simulink model "final_model16b"  (Simulink 8.8)
settings: Solver=ode5  StartTime=0.0  StopTime=0.8  FixedStep=1e-06  RelTol=1e-3
undefined symbols (not defined in the file or in its folder): Acid, Lead
libraries: spsCurrentMeasurementLib x14, spsSeriesRLCBranchLib x12, simulink x9, spsVoltageMeasurementLib x9, spsIGBTDiodeLib x6, spsDiodeLib x5, spsParallelRLCBranchLib x4, spsMosfetLib x2, spsAlphaBetaZerotodq0Lib x2, spsBatteryLib x1, spspowerguiLib x1, spsThreePhaseVIMeasurementLib x1
settings Model: Creator=Aditya  LastModifiedBy=Aditya
settings DataIOCC: LimitDataPoints=off  SaveFormat=Dataset  SignalLoggingSaveFormat=Dataset  ReturnWorkspaceOutputs=on
settings OptimizationCC: LifeSpan=auto
settings DebuggingCC: UnderspecifiedInitializationDetection=Simplified  MergeDetectMultiDrivingBlocksExec=error  FcnCallInpInsideContextMsg=error  StateNameClashWarn=none  SFUnexpectedBacktrackingDiag=error  SFNoUnconditionalDefaultTransitionDiag=error  SFExecutionAtInitializationDiag=warning  SFMachineParentedDataDiag=error
settings HardwareCC: ProdBitPerPointer=64  ProdBitPerSizeT=64  ProdBitPerPtrDiffT=64  ProdLargestAtomicFloat=Float  ProdIntDivRoundTo=Zero  ProdEndianess=LittleEndian  ProdWordSize=64  ProdHWDeviceType=Intel->x86-64 (Windows64)
settings ModelReferenceCC: PropagateSignalLabelsOutOfModel=on
settings SFSimCC: SimUseLocalCustomCode=on
settings RTWCC: RTWUseLocalCustomCode=on
settings GRTTargetCC: TargetLangStandard=C99 (ISO)  CombineOutputUpdateFcns=on  GRTInterface=off
settings ConfigComp: CovMetricSettings=dwe  CovSaveCumulativeToWorkspaceVar=off  CovSaveSingleToWorkspaceVar=off  CovExternalEMLEnable=on

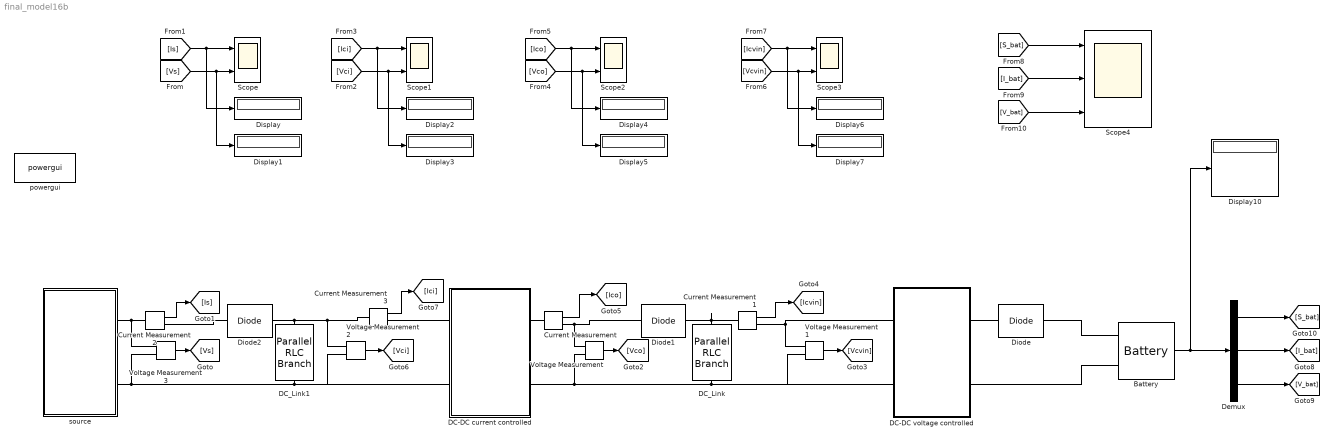
== system final_model16b ==
  Battery : spsBatteryLib/Battery  BatType=Lead-Acid  ShowTempParam=off  ThermalPreset=no  ShowAgeParam=off  NomV=48  NomQ=150  SOC=50  Batt_Tr=0.1  PresetModel=on  MaxQ=156.25  MinV=36  FullV=52.2632  Dis_rate=30  R=0.0032  Normal_OP=46.5417  expZone="[48.8684          0.5]"  current=[6.5 13 32.5]  Units=Time  Tci=20  NomT=20  T2=-30  MaxQ2=4.8  FullV2=7.1  Normal_OP2=5.655  expZone2="[6.58           1]"  Rca=0.6  ti=2000  Dp=0  Neq0=0  Tsim=1e6  Ta1=25  Qeol=5.4*0.9  Reol=0.013333*1.2  Char_age=[2.3478, 3]  Dis_age=[2.3478, 10]  N1=1500  N2=10500  N3=1000  N4=1400  Ta2=45  N5=950
  Current Measurement{,1..3} (4 alike) : spsCurrentMeasurementLib/Current Measurement  PhasorSimulation=off  OutputType=Complex  PSBequivalent=0
  DC-DC current controlled : Subsystem
  DC-DC voltage controlled : Subsystem
  DC_Link : spsParallelRLCBranchLib/Parallel RLC Branch  LConnTagsString=a  RConnTagsString=__new0  BranchType=C  Resistance=1  Inductance=1e-3  SetiL0=off  InitialCurrent=0  Capacitance=300e-6  Setx0=off  InitialVoltage=0  Measurements=None
  DC_Link1 : spsParallelRLCBranchLib/Parallel RLC Branch  LConnTagsString=a  RConnTagsString=__new0  BranchType=C  Resistance=1  Inductance=1e-3  SetiL0=off  InitialCurrent=0  Capacitance=300e-6  Setx0=off  InitialVoltage=0  Measurements=None
  Demux : Demux  Outputs=3
  Diode : spsDiodeLib/Diode  Ron=0.001  Lon=0  Vf=0.8  IC=0  UseSnubber=0  Rs=500  Cs=250e-9  Measurements=off
  Diode1 : spsDiodeLib/Diode  Ron=0.001  Lon=0  Vf=0.8  IC=0  UseSnubber=0  Rs=500  Cs=250e-9  Measurements=off
  Diode2 : spsDiodeLib/Diode  Ron=0.001  Lon=0  Vf=0.8  IC=0  UseSnubber=0  Rs=500  Cs=250e-9  Measurements=off
  Display{,1..7,10} (9 alike) : Display
  Scope{,1..3} (4 alike) : Scope  NumInputPorts=2
  Scope4 : Scope  NumInputPorts=3
  Voltage Measurement{,1..3} (4 alike) : spsVoltageMeasurementLib/Voltage Measurement  PhasorSimulation=off  OutputType=Complex  PSBequivalent=0
  powergui : spspowerguiLib/powergui  Priority=1  SimulationMode=Discrete  SampleTime=1e-06  frequency=60  Iterations=50  frequencyindice=0  Pbase=100e6  ErrMax=1e-4  UnitsV=kV  UnitsW=MW  buscounter=0  FunctionMessages=off  echomessages=off  EnableUseOfTLC=off  CurrentSourceSwitches=off  DisableSnubberDevices=off  DisableRonSwitches=off  DisableVfSwitches=off  DisplayEquations=off  AutomaticDiscreteSolvers=off  SolverType=Tustin/Backward Euler (TBE)  Interpol=off  ExternalGateDelay=off  methode=off  Ts=100  x0status=blocks  SPID=on  SwTol=0  HookPort=off  NonlinearTolerance=1e-4  nMaxIteration=100  ContinueOnMaxIteration=off  RestoreLinks=warning  ResistiveCurrentMeasurement=off  Frange=[0:2:500]  Ylog=off  Xlog=on  ShowGrid=off  save=off  variable=ZData  structure=0  ZoomFFT=off  StartTime=0.0  cycles=1  DisplayStyle=1  fundamental=60  FreqAxis=off  MaxFrequency=1000  frequencyindicesteady=1  RmsSteady=1  display=off
  source : Subsystem
  wires:
  Voltage Measurement3/1 -> [Vs]
  Current Measurement2/1 -> [Is]
  Voltage Measurement/1 -> [Vco]
  Voltage Measurement1/1 -> [Vcvin]
  Current Measurement/1 -> [Ico]
  Current Measurement1/1 -> [Icvin]
  Voltage Measurement2/1 -> [Vci]
  Current Measurement3/1 -> [Ici]
  [Is] -> Display/1, Scope/1
  [Vs] -> Display1/1, Scope/2
  [Vci] -> Display3/1, Scope1/2
  [Ici] -> Display2/1, Scope1/1
  [Vco] -> Display5/1, Scope2/2
  [Ico] -> Display4/1, Scope2/1
  [Vcvin] -> Display7/1, Scope3/2
  [Icvin] -> Display6/1, Scope3/1
  Battery/1 -> Demux/1, Display10/1
  Demux/1 -> [S_bat]
  Demux/2 -> [I_bat]
  Demux/3 -> [V_bat]
  [S_bat] -> Scope4/1
  [I_bat] -> Scope4/2
  [V_bat] -> Scope4/3
  connections:
  Current Measurement3/LConn1 -- Diode2/RConn1 -- DC_Link1/LConn1 -- Voltage Measurement2/LConn1
  source/LConn2 -- Voltage Measurement3/LConn2 -- Voltage Measurement2/LConn2 -- DC-DC current controlled/LConn2 -- DC_Link1/RConn1
  Current Measurement/RConn1 -- Diode1/LConn1 -- Voltage Measurement/LConn1
  DC-DC current controlled/RConn2 -- Voltage Measurement/LConn2 -- Voltage Measurement1/LConn2 -- DC-DC voltage controlled/LConn2 -- DC_Link/RConn1
  Current Measurement/LConn1 -- DC-DC current controlled/RConn1
  Voltage Measurement1/LConn1 -- Current Measurement1/RConn1 -- DC-DC voltage controlled/LConn1
  Current Measurement3/RConn1 -- DC-DC current controlled/LConn1
  Current Measurement2/LConn1 -- Voltage Measurement3/LConn1 -- source/LConn1
  Diode/LConn1 -- DC-DC voltage controlled/RConn1
  Battery/LConn2 -- DC-DC voltage controlled/RConn2
  Battery/LConn1 -- Diode/RConn1
  DC_Link/LConn1 -- Diode1/RConn1 -- Current Measurement1/LConn1
  Current Measurement2/RConn1 -- Diode2/LConn1

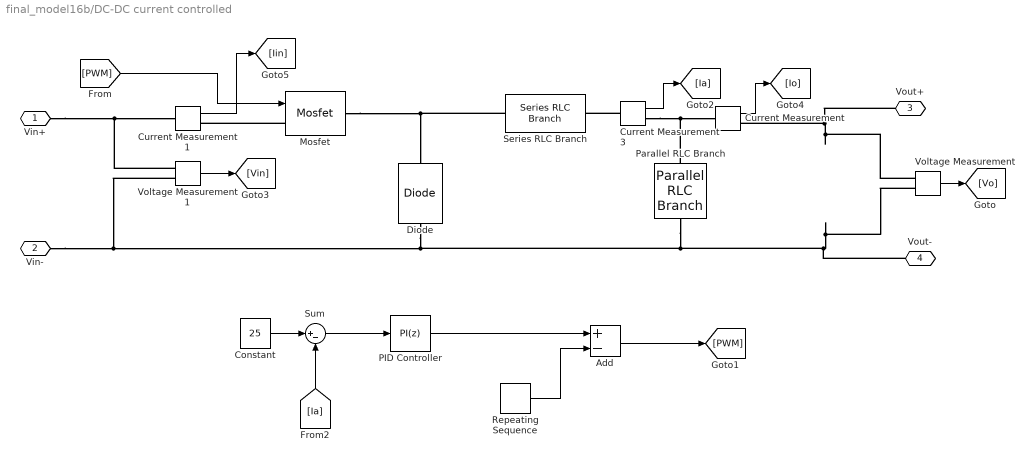
== system final_model16b/DC-DC current controlled ==
  Add : Sum  Inputs=+-
  Constant : Constant  Value=25
  Current Measurement : spsCurrentMeasurementLib/Current Measurement  PhasorSimulation=off  OutputType=Complex  PSBequivalent=0
  Current Measurement1 : spsCurrentMeasurementLib/Current Measurement  PhasorSimulation=off  OutputType=Complex  PSBequivalent=0
  Current Measurement3 : spsCurrentMeasurementLib/Current Measurement  PhasorSimulation=off  OutputType=Complex  PSBequivalent=0
  Diode : spsDiodeLib/Diode  Ron=0.001  Lon=0  Vf=0.8  IC=0  UseSnubber=0  Rs=500  Cs=250e-9  Measurements=off
  Mosfet : spsMosfetLib/Mosfet  Ron=0.1  Lon=0  Rd=0.01  Vfd=0  IC=0  Rs=1e5  Cs=inf  Measurements=off
  PID Controller : simulink/Continuous/PID Controller  Controller=PI  Form=Parallel  TimeDomain=Discrete-time  SampleTime=-1  IntegratorMethod=Forward Euler  ControllerParametersSource=internal  P=0.4928  I=0.93  D=0  UseFilter=on  N=100  InitialConditionSource=internal  InitialConditionForIntegrator=0  InitialConditionForFilter=0  DifferentiatorICPrevScaledInput=0  ExternalReset=none  TrackingMode=off  Kt=1  LimitOutput=off  UpperSaturationLimit=inf  LowerSaturationLimit=-inf  LinearizeAsGain=on  AntiWindupMode=none  Kb=1  POutMin=[]  POutMax=[]  IOutMin=[]  IOutMax=[]  DOutMin=[]  DOutMax=[]  NOutMin=[]  NOutMax=[]  SumOutMin=[]  SumOutMax=[]  SaturationOutMin=[]  SaturationOutMax=[]  PParamMin=[]  PParamMax=[]  IParamMin=[]  IParamMax=[]  DParamMin=[]  DParamMax=[]  NParamMin=[]  NParamMax=[]  KbParamMin=[]  KbParamMax=[]  KtParamMin=[]  KtParamMax=[]  KbOutMin=[]  KbOutMax=[]  KtOutMin=[]  KtOutMax=[]  IntegratorOutMin=[]  IntegratorOutMax=[]  FilterOutMin=[]  FilterOutMax=[]  SumI1OutMin=[]  SumI1OutMax=[]  SumI2OutMin=[]  SumI2OutMax=[]  SumI3OutMin=[]  SumI3OutMax=[]  SumDOutMin=[]  SumDOutMax=[]  DifferentiatorOutMin=[]  DifferentiatorOutMax=[]  IntegratorContinuousStateAttributes=''  IntegratorStateMustResolveToSignalObject=off  IntegratorRTWStateStorageClass=Auto  FilterContinuousStateAttributes=''  FilterStateMustResolveToSignalObject=off  FilterRTWStateStorageClass=Auto
  Parallel RLC Branch : spsParallelRLCBranchLib/Parallel RLC Branch  LConnTagsString=a  RConnTagsString=__new0  BranchType=C  Resistance=1  Inductance=1e-3  SetiL0=off  InitialCurrent=0  Capacitance=20e-6  Setx0=off  InitialVoltage=0  Measurements=None
  Repeating Sequence : simulink/Sources/Repeating Sequence  rep_seq_t=[0 0.25/2000 0.5/2000 0.75/2000 1/2000]  rep_seq_y=[0 -1 0 1 0]
  Series RLC Branch : spsSeriesRLCBranchLib/Series RLC Branch  LConnTagsString=__new0  RConnTagsString=__new0  BranchType=L  Resistance=10  Inductance=0.01  SetiL0=off  InitialCurrent=0  Capacitance=1e-6  Setx0=off  InitialVoltage=0  Measurements=None
  Sum : Sum  Inputs=|+-
  Voltage Measurement : spsVoltageMeasurementLib/Voltage Measurement  PhasorSimulation=off  OutputType=Complex  PSBequivalent=0
  Voltage Measurement1 : spsVoltageMeasurementLib/Voltage Measurement  PhasorSimulation=off  OutputType=Complex  PSBequivalent=0
  Vin+ : PMIOPort  Side=Left
  Vin- : PMIOPort  Port=2  Side=Left
  Vout+ : PMIOPort  Port=3  Side=Right
  Vout- : PMIOPort  Port=4  Side=Right
  wires:
  Sum/1 -> PID Controller/1
  Voltage Measurement1/1 -> [Vin]
  [PWM] -> Mosfet/1
  Constant/1 -> Sum/1
  PID Controller/1 -> Add/1
  Add/1 -> [PWM]
  Repeating Sequence/1 -> Add/2
  [Ia] -> Sum/2
  Current Measurement3/1 -> [Ia]
  Voltage Measurement/1 -> [Vo]
  Current Measurement/1 -> [Io]
  Current Measurement1/1 -> [Iin]
  connections:
  Mosfet/RConn1 -- Diode/RConn1 -- Series RLC Branch/LConn1
  Voltage Measurement1/LConn2 -- Vin-/RConn1 -- Voltage Measurement/LConn2 -- Vout-/RConn1 -- Parallel RLC Branch/RConn1 -- Diode/LConn1
  Parallel RLC Branch/LConn1 -- Current Measurement/LConn1 -- Current Measurement3/RConn1
  Mosfet/LConn1 -- Current Measurement1/RConn1
  Vout+/RConn1 -- Current Measurement/RConn1 -- Voltage Measurement/LConn1
  Voltage Measurement1/LConn1 -- Vin+/RConn1 -- Current Measurement1/LConn1
  Current Measurement3/LConn1 -- Series RLC Branch/RConn1

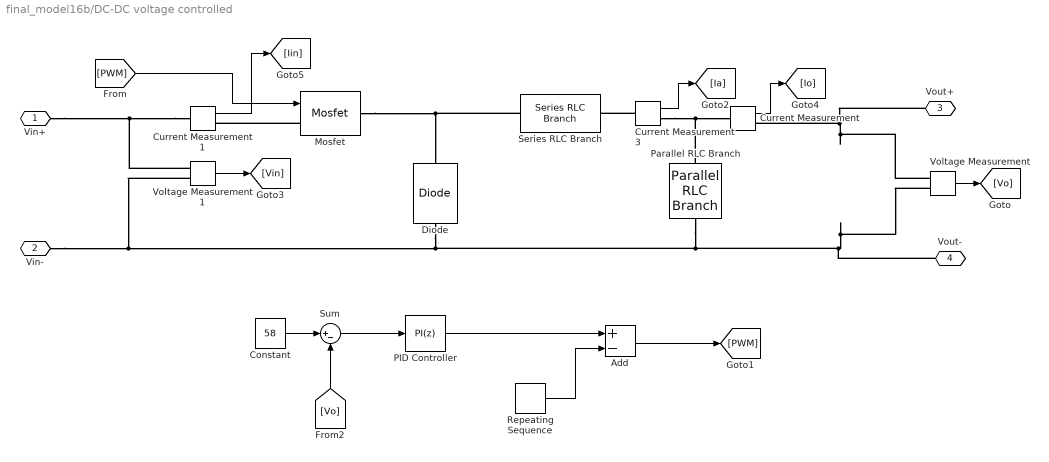
== system final_model16b/DC-DC voltage controlled ==
  Add : Sum  Inputs=+-
  Constant : Constant  Value=58
  Current Measurement : spsCurrentMeasurementLib/Current Measurement  PhasorSimulation=off  OutputType=Complex  PSBequivalent=0
  Current Measurement1 : spsCurrentMeasurementLib/Current Measurement  PhasorSimulation=off  OutputType=Complex  PSBequivalent=0
  Current Measurement3 : spsCurrentMeasurementLib/Current Measurement  PhasorSimulation=off  OutputType=Complex  PSBequivalent=0
  Diode : spsDiodeLib/Diode  Ron=0.001  Lon=0  Vf=0.8  IC=0  UseSnubber=0  Rs=500  Cs=250e-9  Measurements=off
  Mosfet : spsMosfetLib/Mosfet  Ron=0.1  Lon=0  Rd=0.01  Vfd=0  IC=0  Rs=1e5  Cs=inf  Measurements=off
  PID Controller : simulink/Continuous/PID Controller  Controller=PI  Form=Parallel  TimeDomain=Discrete-time  SampleTime=-1  IntegratorMethod=Forward Euler  ControllerParametersSource=internal  P=0.4928  I=0.93  D=0  UseFilter=on  N=100  InitialConditionSource=internal  InitialConditionForIntegrator=0  InitialConditionForFilter=0  DifferentiatorICPrevScaledInput=0  ExternalReset=none  TrackingMode=off  Kt=1  LimitOutput=off  UpperSaturationLimit=inf  LowerSaturationLimit=-inf  LinearizeAsGain=on  AntiWindupMode=none  Kb=1  POutMin=[]  POutMax=[]  IOutMin=[]  IOutMax=[]  DOutMin=[]  DOutMax=[]  NOutMin=[]  NOutMax=[]  SumOutMin=[]  SumOutMax=[]  SaturationOutMin=[]  SaturationOutMax=[]  PParamMin=[]  PParamMax=[]  IParamMin=[]  IParamMax=[]  DParamMin=[]  DParamMax=[]  NParamMin=[]  NParamMax=[]  KbParamMin=[]  KbParamMax=[]  KtParamMin=[]  KtParamMax=[]  KbOutMin=[]  KbOutMax=[]  KtOutMin=[]  KtOutMax=[]  IntegratorOutMin=[]  IntegratorOutMax=[]  FilterOutMin=[]  FilterOutMax=[]  SumI1OutMin=[]  SumI1OutMax=[]  SumI2OutMin=[]  SumI2OutMax=[]  SumI3OutMin=[]  SumI3OutMax=[]  SumDOutMin=[]  SumDOutMax=[]  DifferentiatorOutMin=[]  DifferentiatorOutMax=[]  IntegratorContinuousStateAttributes=''  IntegratorStateMustResolveToSignalObject=off  IntegratorRTWStateStorageClass=Auto  FilterContinuousStateAttributes=''  FilterStateMustResolveToSignalObject=off  FilterRTWStateStorageClass=Auto
  Parallel RLC Branch : spsParallelRLCBranchLib/Parallel RLC Branch  LConnTagsString=a  RConnTagsString=__new0  BranchType=C  Resistance=1  Inductance=1e-3  SetiL0=off  InitialCurrent=0  Capacitance=20e-6  Setx0=off  InitialVoltage=0  Measurements=None
  Repeating Sequence : simulink/Sources/Repeating Sequence  rep_seq_t=[0 0.25/2000 0.5/2000 0.75/2000 1/2000]  rep_seq_y=[0 -1 0 1 0]
  Series RLC Branch : spsSeriesRLCBranchLib/Series RLC Branch  LConnTagsString=__new0  RConnTagsString=__new0  BranchType=L  Resistance=10  Inductance=0.01  SetiL0=off  InitialCurrent=0  Capacitance=1e-6  Setx0=off  InitialVoltage=0  Measurements=None
  Sum : Sum  Inputs=|+-
  Voltage Measurement : spsVoltageMeasurementLib/Voltage Measurement  PhasorSimulation=off  OutputType=Complex  PSBequivalent=0
  Voltage Measurement1 : spsVoltageMeasurementLib/Voltage Measurement  PhasorSimulation=off  OutputType=Complex  PSBequivalent=0
  Vin+ : PMIOPort  Side=Left
  Vin- : PMIOPort  Port=2  Side=Left
  Vout+ : PMIOPort  Port=3  Side=Right
  Vout- : PMIOPort  Port=4  Side=Right
  wires:
  Constant/1 -> Sum/1
  Repeating Sequence/1 -> Add/2
  Current Measurement/1 -> [Io]
  Add/1 -> [PWM]
  PID Controller/1 -> Add/1
  [PWM] -> Mosfet/1
  Voltage Measurement/1 -> [Vo]
  Current Measurement3/1 -> [Ia]
  [Vo] -> Sum/2
  Sum/1 -> PID Controller/1
  Voltage Measurement1/1 -> [Vin]
  Current Measurement1/1 -> [Iin]
  connections:
  Current Measurement3/LConn1 -- Series RLC Branch/RConn1
  Mosfet/RConn1 -- Diode/RConn1 -- Series RLC Branch/LConn1
  Current Measurement3/RConn1 -- Current Measurement/LConn1 -- Parallel RLC Branch/LConn1
  Vout+/RConn1 -- Current Measurement/RConn1 -- Voltage Measurement/LConn1
  Diode/LConn1 -- Vin-/RConn1 -- Voltage Measurement1/LConn2 -- Voltage Measurement/LConn2 -- Vout-/RConn1 -- Parallel RLC Branch/RConn1
  Current Measurement1/LConn1 -- Vin+/RConn1 -- Voltage Measurement1/LConn1
  Mosfet/LConn1 -- Current Measurement1/RConn1

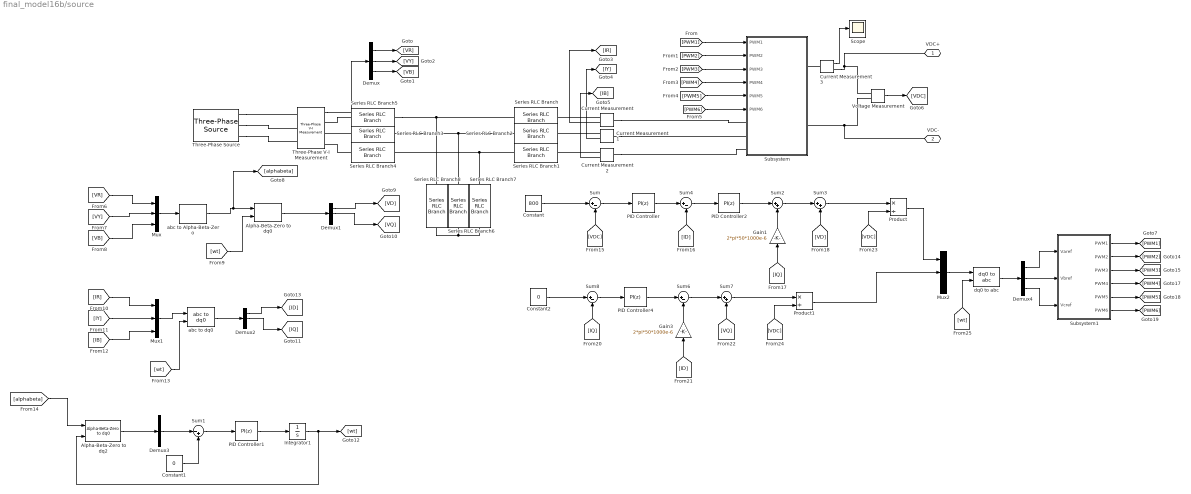
== system final_model16b/source ==
  Alpha-Beta-Zero to dq0 : spsAlphaBetaZerotodq0Lib/Alpha-Beta-Zero to dq0  Alignment=90 degrees behind phase A axis
  Alpha-Beta-Zero to dq2 : spsAlphaBetaZerotodq0Lib/Alpha-Beta-Zero to dq0  Alignment=90 degrees behind phase A axis
  Constant : Constant  Value=800
  Constant1 : Constant  Value=0
  Constant2 : Constant  Value=0
  Current Measurement{,1..3} (4 alike) : spsCurrentMeasurementLib/Current Measurement  PhasorSimulation=off  OutputType=Complex  PSBequivalent=0
  Demux{,1..4} (5 alike) : Demux  Outputs=3
  Gain1 : Gain  Gain=2*pi*50*1000e-6
  Gain3 : Gain  Gain=2*pi*50*1000e-6
  Integrator1 : Integrator
  Mux : Mux  Inputs=3
  Mux1 : Mux  Inputs=3
  Mux2 : Mux  Inputs=3
  PID Controller : simulink/Continuous/PID Controller  Controller=PI  Form=Parallel  TimeDomain=Discrete-time  SampleTime=-1  IntegratorMethod=Forward Euler  ControllerParametersSource=internal  P=0.5  I=200  D=0  UseFilter=on  N=100  InitialConditionSource=internal  InitialConditionForIntegrator=0  InitialConditionForFilter=0  DifferentiatorICPrevScaledInput=0  ExternalReset=none  TrackingMode=off  Kt=1  LimitOutput=off  UpperSaturationLimit=inf  LowerSaturationLimit=-inf  LinearizeAsGain=on  AntiWindupMode=none  Kb=1  POutMin=[]  POutMax=[]  IOutMin=[]  IOutMax=[]  DOutMin=[]  DOutMax=[]  NOutMin=[]  NOutMax=[]  SumOutMin=[]  SumOutMax=[]  SaturationOutMin=[]  SaturationOutMax=[]  PParamMin=[]  PParamMax=[]  IParamMin=[]  IParamMax=[]  DParamMin=[]  DParamMax=[]  NParamMin=[]  NParamMax=[]  KbParamMin=[]  KbParamMax=[]  KtParamMin=[]  KtParamMax=[]  KbOutMin=[]  KbOutMax=[]  KtOutMin=[]  KtOutMax=[]  IntegratorOutMin=[]  IntegratorOutMax=[]  FilterOutMin=[]  FilterOutMax=[]  SumI1OutMin=[]  SumI1OutMax=[]  SumI2OutMin=[]  SumI2OutMax=[]  SumI3OutMin=[]  SumI3OutMax=[]  SumDOutMin=[]  SumDOutMax=[]  DifferentiatorOutMin=[]  DifferentiatorOutMax=[]  IntegratorContinuousStateAttributes=''  IntegratorStateMustResolveToSignalObject=off  IntegratorRTWStateStorageClass=Auto  FilterContinuousStateAttributes=''  FilterStateMustResolveToSignalObject=off  FilterRTWStateStorageClass=Auto
  PID Controller1 : simulink/Continuous/PID Controller  Controller=PI  Form=Parallel  TimeDomain=Discrete-time  SampleTime=-1  IntegratorMethod=Forward Euler  ControllerParametersSource=internal  P=1  I=1  D=0  UseFilter=on  N=100  InitialConditionSource=internal  InitialConditionForIntegrator=0  InitialConditionForFilter=0  DifferentiatorICPrevScaledInput=0  ExternalReset=none  TrackingMode=off  Kt=1  LimitOutput=off  UpperSaturationLimit=inf  LowerSaturationLimit=-inf  LinearizeAsGain=on  AntiWindupMode=none  Kb=1  POutMin=[]  POutMax=[]  IOutMin=[]  IOutMax=[]  DOutMin=[]  DOutMax=[]  NOutMin=[]  NOutMax=[]  SumOutMin=[]  SumOutMax=[]  SaturationOutMin=[]  SaturationOutMax=[]  PParamMin=[]  PParamMax=[]  IParamMin=[]  IParamMax=[]  DParamMin=[]  DParamMax=[]  NParamMin=[]  NParamMax=[]  KbParamMin=[]  KbParamMax=[]  KtParamMin=[]  KtParamMax=[]  KbOutMin=[]  KbOutMax=[]  KtOutMin=[]  KtOutMax=[]  IntegratorOutMin=[]  IntegratorOutMax=[]  FilterOutMin=[]  FilterOutMax=[]  SumI1OutMin=[]  SumI1OutMax=[]  SumI2OutMin=[]  SumI2OutMax=[]  SumI3OutMin=[]  SumI3OutMax=[]  SumDOutMin=[]  SumDOutMax=[]  DifferentiatorOutMin=[]  DifferentiatorOutMax=[]  IntegratorContinuousStateAttributes=''  IntegratorStateMustResolveToSignalObject=off  IntegratorRTWStateStorageClass=Auto  FilterContinuousStateAttributes=''  FilterStateMustResolveToSignalObject=off  FilterRTWStateStorageClass=Auto
  PID Controller2 : simulink/Continuous/PID Controller  Controller=PI  Form=Parallel  TimeDomain=Discrete-time  SampleTime=-1  IntegratorMethod=Forward Euler  ControllerParametersSource=internal  P=25  I=500  D=0  UseFilter=on  N=100  InitialConditionSource=internal  InitialConditionForIntegrator=0  InitialConditionForFilter=0  DifferentiatorICPrevScaledInput=0  ExternalReset=none  TrackingMode=off  Kt=1  LimitOutput=off  UpperSaturationLimit=inf  LowerSaturationLimit=-inf  LinearizeAsGain=on  AntiWindupMode=none  Kb=1  POutMin=[]  POutMax=[]  IOutMin=[]  IOutMax=[]  DOutMin=[]  DOutMax=[]  NOutMin=[]  NOutMax=[]  SumOutMin=[]  SumOutMax=[]  SaturationOutMin=[]  SaturationOutMax=[]  PParamMin=[]  PParamMax=[]  IParamMin=[]  IParamMax=[]  DParamMin=[]  DParamMax=[]  NParamMin=[]  NParamMax=[]  KbParamMin=[]  KbParamMax=[]  KtParamMin=[]  KtParamMax=[]  KbOutMin=[]  KbOutMax=[]  KtOutMin=[]  KtOutMax=[]  IntegratorOutMin=[]  IntegratorOutMax=[]  FilterOutMin=[]  FilterOutMax=[]  SumI1OutMin=[]  SumI1OutMax=[]  SumI2OutMin=[]  SumI2OutMax=[]  SumI3OutMin=[]  SumI3OutMax=[]  SumDOutMin=[]  SumDOutMax=[]  DifferentiatorOutMin=[]  DifferentiatorOutMax=[]  IntegratorContinuousStateAttributes=''  IntegratorStateMustResolveToSignalObject=off  IntegratorRTWStateStorageClass=Auto  FilterContinuousStateAttributes=''  FilterStateMustResolveToSignalObject=off  FilterRTWStateStorageClass=Auto
  PID Controller4 : simulink/Continuous/PID Controller  Controller=PI  Form=Parallel  TimeDomain=Discrete-time  SampleTime=-1  IntegratorMethod=Forward Euler  ControllerParametersSource=internal  P=25  I=500  D=0  UseFilter=on  N=100  InitialConditionSource=internal  InitialConditionForIntegrator=0  InitialConditionForFilter=0  DifferentiatorICPrevScaledInput=0  ExternalReset=none  TrackingMode=off  Kt=1  LimitOutput=off  UpperSaturationLimit=inf  LowerSaturationLimit=-inf  LinearizeAsGain=on  AntiWindupMode=none  Kb=1  POutMin=[]  POutMax=[]  IOutMin=[]  IOutMax=[]  DOutMin=[]  DOutMax=[]  NOutMin=[]  NOutMax=[]  SumOutMin=[]  SumOutMax=[]  SaturationOutMin=[]  SaturationOutMax=[]  PParamMin=[]  PParamMax=[]  IParamMin=[]  IParamMax=[]  DParamMin=[]  DParamMax=[]  NParamMin=[]  NParamMax=[]  KbParamMin=[]  KbParamMax=[]  KtParamMin=[]  KtParamMax=[]  KbOutMin=[]  KbOutMax=[]  KtOutMin=[]  KtOutMax=[]  IntegratorOutMin=[]  IntegratorOutMax=[]  FilterOutMin=[]  FilterOutMax=[]  SumI1OutMin=[]  SumI1OutMax=[]  SumI2OutMin=[]  SumI2OutMax=[]  SumI3OutMin=[]  SumI3OutMax=[]  SumDOutMin=[]  SumDOutMax=[]  DifferentiatorOutMin=[]  DifferentiatorOutMax=[]  IntegratorContinuousStateAttributes=''  IntegratorStateMustResolveToSignalObject=off  IntegratorRTWStateStorageClass=Auto  FilterContinuousStateAttributes=''  FilterStateMustResolveToSignalObject=off  FilterRTWStateStorageClass=Auto
  Product : Product  Inputs=*/
  Product1 : Product  Inputs=*/
  Scope : Scope
  Series RLC Branch{,1..5} (6 alike) : spsSeriesRLCBranchLib/Series RLC Branch  LConnTagsString=__new0  RConnTagsString=__new0  BranchType=L  Resistance=1  Inductance=500e-6  SetiL0=off  InitialCurrent=0  Capacitance=1e-6  Setx0=off  InitialVoltage=0  Measurements=None
  Series RLC Branch6 : spsSeriesRLCBranchLib/Series RLC Branch  LConnTagsString=__new0  RConnTagsString=__new0  BranchType=C  Resistance=1  Inductance=1e-3  SetiL0=off  InitialCurrent=0  Capacitance=100e-6  Setx0=off  InitialVoltage=0  Measurements=None
  Series RLC Branch7 : spsSeriesRLCBranchLib/Series RLC Branch  LConnTagsString=__new0  RConnTagsString=__new0  BranchType=C  Resistance=1  Inductance=1e-3  SetiL0=off  InitialCurrent=0  Capacitance=100e-6  Setx0=off  InitialVoltage=0  Measurements=None
  Series RLC Branch8 : spsSeriesRLCBranchLib/Series RLC Branch  LConnTagsString=__new0  RConnTagsString=__new0  BranchType=C  Resistance=1  Inductance=1e-3  SetiL0=off  InitialCurrent=0  Capacitance=100e-6  Setx0=off  InitialVoltage=0  Measurements=None
  Subsystem : Subsystem
  Subsystem1 : Subsystem
  Sum{,4,6,8} (4 alike) : Sum  Inputs=|+-
  Sum1 : Sum  Inputs=|-+
  Sum2 : Sum  Inputs=|++
  Sum3 : Sum  Inputs=|++
  Sum7 : Sum  Inputs=|++
  Three-Phase V-I Measurement : spsThreePhaseVIMeasurementLib/Three-Phase V-I Measurement  VoltageMeasurement=phase-to-phase  SetLabelV=off  LabelV=Vabc  Vpu=off  VpuLL=off  CurrentMeasurement=no  SetLabelI=off  LabelI=Iabc  Ipu=off  Pbase=100e6  Vbase=500e3  OutputType=Complex  PhasorSimulation=off  PSBequivalent=0
  Three-Phase Source : spsThreePhaseSourceLib/Three-Phase Source  InternalConnection=Yg  VoltagePhases=off  Voltage=415  PhaseAngle=0  Voltage_phases=[25e3 25e3 25e3]/sqrt(3)  PhaseAngles_phases=[0 -120 +120]  Frequency=50  NonIdealSource=on  SpecifyImpedance=on  Resistance=0.8929e-3  Inductance=16.58e-9  ShortCircuitLevel=inf  BaseVoltage=415  XRratio=7  BusType=swing  Pref=10e3  Qref=0  Prefabc=[10e3, 10e3, 10e3]  Qrefabc=[0, 0, 0]  Qmin=-inf  Qmax=inf
  Voltage Measurement : spsVoltageMeasurementLib/Voltage Measurement  PhasorSimulation=off  OutputType=Complex  PSBequivalent=0
  abc to Alpha-Beta-Zero : spsabctoAlphaBetaZeroLib/abc to Alpha-Beta-Zero
  abc to dq0 : spsabctodq0Lib/abc to dq0  Alignment=90 degrees behind phase A axis
  dq0 to abc : spsdq0toabcLib/dq0 to abc  Alignment=90 degrees behind phase A axis
  VDC+ : PMIOPort  Side=Left
  VDC- : PMIOPort  Port=2  Side=Left
  wires:
  [PWM6] -> Subsystem/6(PWM6)
  Demux/1 -> [VR]
  [ID] -> Gain3/1
  Constant/1 -> Sum/1
  Demux/2 -> [VY]
  PID Controller1/1 -> Integrator1/1
  Voltage Measurement/1 -> [VDC]
  abc to Alpha-Beta-Zero/1 -> [alphabeta], Alpha-Beta-Zero to dq0/1
  Demux2/2 -> [IQ]
  PID Controller4/1 -> Sum6/1
  Current Measurement/1 -> [IR]
  Subsystem1/1(PWM1) -> [PWM1]
  Subsystem1/3(PWM3) -> [PWM3]
  [VR] -> Mux/1
  [ID] -> Sum4/2
  [PWM4] -> Subsystem/4(PWM4)
  Current Measurement2/1 -> [IB]
  Alpha-Beta-Zero to dq2/1 -> Demux3/1
  [IY] -> Mux1/2
  [VDC] -> Sum/2
  [wt] -> Alpha-Beta-Zero to dq0/2
  [PWM2] -> Subsystem/2(PWM2)
  [PWM5] -> Subsystem/5(PWM5)
  Three-Phase V-I Measurement/1 -> Demux/1
  Sum3/1 -> Product/1
  Constant1/1 -> Sum1/2
  [VY] -> Mux/2
  Subsystem1/4(PWM4) -> [PWM4]
  Alpha-Beta-Zero to dq0/1 -> Demux1/1
  Demux1/1 -> [VD]
  Sum4/1 -> PID Controller2/1
  Integrator1/1 -> [wt], Alpha-Beta-Zero to dq2/2
  dq0 to abc/1 -> Demux4/1
  Demux1/2 -> [VQ]
  [wt] -> dq0 to abc/2
  [IR] -> Mux1/1
  Demux3/2 -> Sum1/1
  Current Measurement1/1 -> [IY]
  Demux/3 -> [VB]
  Subsystem1/6(PWM6) -> [PWM6]
  Gain3/1 -> Sum6/2
  [PWM3] -> Subsystem/3(PWM3)
  Subsystem1/2(PWM2) -> [PWM2]
  [VD] -> Sum3/2
  PID Controller2/1 -> Sum2/1
  [VB] -> Mux/3
  PID Controller/1 -> Sum4/1
  Gain1/1 -> Sum2/2
  Sum2/1 -> Sum3/1
  [wt] -> abc to dq0/2
  Subsystem1/5(PWM5) -> [PWM5]
  [VQ] -> Sum7/2
  [alphabeta] -> Alpha-Beta-Zero to dq2/1
  [IB] -> Mux1/3
  abc to dq0/1 -> Demux2/1
  [PWM1] -> Subsystem/1(PWM1)
  Demux2/1 -> [ID]
  Mux1/1 -> abc to dq0/1
  Sum6/1 -> Sum7/1
  Sum7/1 -> Product1/1
  Mux2/1 -> dq0 to abc/1
  Sum/1 -> PID Controller/1
  [VDC] -> Product1/2
  Mux/1 -> abc to Alpha-Beta-Zero/1
  Product1/1 -> Mux2/2
  Product/1 -> Mux2/1
  [IQ] -> Gain1/1
  [VDC] -> Product/2
  [IQ] -> Sum8/2
  Constant2/1 -> Sum8/1
  Demux4/2 -> Subsystem1/2(Vbref)
  Sum8/1 -> PID Controller4/1
  Demux4/1 -> Subsystem1/1(Varef)
  Sum1/1 -> PID Controller1/1
  Demux4/3 -> Subsystem1/3(Vcref)
  Current Measurement3/1 -> Scope/1
  connections:
  Current Measurement3/RConn1 -- Voltage Measurement/LConn1 -- VDC+/RConn1
  Series RLC Branch8/RConn1 -- Series RLC Branch6/RConn1 -- Series RLC Branch7/RConn1
  Series RLC Branch2/LConn1 -- Series RLC Branch3/RConn1 -- Series RLC Branch6/LConn1
  Voltage Measurement/LConn2 -- Subsystem/RConn2 -- VDC-/RConn1
  Series RLC Branch5/LConn1 -- Three-Phase V-I Measurement/RConn1
  Series RLC Branch5/RConn1 -- Series RLC Branch8/LConn1 -- Series RLC Branch/LConn1
  Series RLC Branch3/LConn1 -- Three-Phase V-I Measurement/RConn2
  Current Measurement/RConn1 -- Series RLC Branch/RConn1
  Current Measurement2/RConn1 -- Series RLC Branch1/RConn1
  Current Measurement1/LConn1 -- Subsystem/LConn2
  Current Measurement1/RConn1 -- Series RLC Branch2/RConn1
  Series RLC Branch1/LConn1 -- Series RLC Branch7/LConn1 -- Series RLC Branch4/RConn1
  Current Measurement2/LConn1 -- Subsystem/LConn3
  Current Measurement/LConn1 -- Subsystem/LConn1
  Current Measurement3/LConn1 -- Subsystem/RConn1
  Three-Phase Source/RConn1 -- Three-Phase V-I Measurement/LConn1
  Three-Phase Source/RConn2 -- Three-Phase V-I Measurement/LConn2
  Series RLC Branch4/LConn1 -- Three-Phase V-I Measurement/RConn3
  Three-Phase Source/RConn3 -- Three-Phase V-I Measurement/LConn3

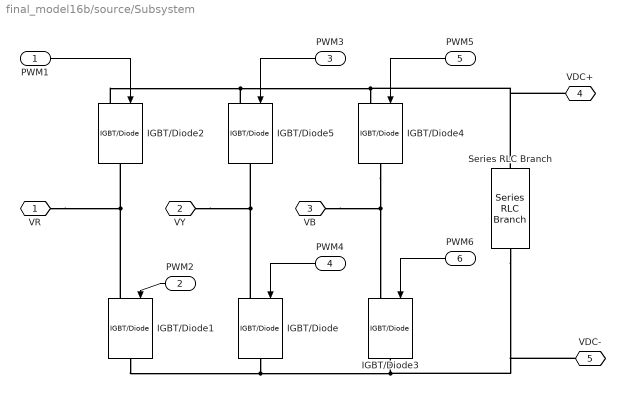
== system final_model16b/source/Subsystem ==
  PWM1 : Inport
  PWM2 : Inport  Port=2
  PWM3 : Inport  Port=3
  PWM4 : Inport  Port=4
  PWM5 : Inport  Port=5
  PWM6 : Inport  Port=6
  IGBT/Diode{,1..5} (6 alike) : spsIGBTDiodeLib/IGBT//Diode  Ron=1e-3  Rs=1e5  Cs=inf  Measurements=off
  Series RLC Branch : spsSeriesRLCBranchLib/Series RLC Branch  LConnTagsString=__new0  RConnTagsString=__new0  BranchType=RC  Resistance=1e-3  Inductance=1e-3  SetiL0=off  InitialCurrent=0  Capacitance=5600e-6  Setx0=off  InitialVoltage=0  Measurements=None
  VR : PMIOPort  Side=Left
  VY : PMIOPort  Port=2  Side=Left
  VB : PMIOPort  Port=3  Side=Left
  VDC+ : PMIOPort  Port=4  Side=Right
  VDC- : PMIOPort  Port=5  Side=Right
  wires:
  PWM1/1 -> IGBT/Diode2/1
  PWM2/1 -> IGBT/Diode1/1
  PWM5/1 -> IGBT/Diode4/1
  PWM6/1 -> IGBT/Diode3/1
  PWM3/1 -> IGBT/Diode5/1
  PWM4/1 -> IGBT/Diode/1
  connections:
  IGBT/Diode/LConn1 -- VY/RConn1 -- IGBT/Diode5/RConn1
  IGBT/Diode1/RConn1 -- IGBT/Diode/RConn1 -- VDC-/RConn1 -- Series RLC Branch/RConn1 -- IGBT/Diode3/RConn1
  IGBT/Diode2/LConn1 -- IGBT/Diode5/LConn1 -- VDC+/RConn1 -- Series RLC Branch/LConn1 -- IGBT/Diode4/LConn1
  IGBT/Diode4/RConn1 -- VB/RConn1 -- IGBT/Diode3/LConn1
  IGBT/Diode1/LConn1 -- VR/RConn1 -- IGBT/Diode2/RConn1

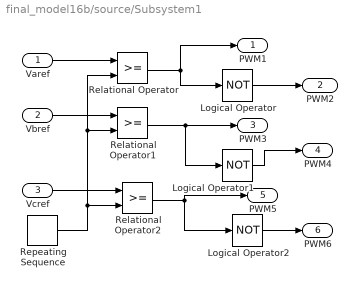
== system final_model16b/source/Subsystem1 ==
  Varef : Inport
  Vbref : Inport  Port=2
  Vcref : Inport  Port=3
  Logical Operator : Logic  Operator=NOT  AllPortsSameDT=off  OutDataTypeStr=boolean
  Logical Operator1 : Logic  Operator=NOT  AllPortsSameDT=off  OutDataTypeStr=boolean
  Logical Operator2 : Logic  Operator=NOT  AllPortsSameDT=off  OutDataTypeStr=boolean
  Relational Operator : RelationalOperator  OutDataTypeStr=boolean  RndMeth=Simplest
  Relational Operator1 : RelationalOperator  OutDataTypeStr=boolean  RndMeth=Simplest
  Relational Operator2 : RelationalOperator  OutDataTypeStr=boolean  RndMeth=Simplest
  Repeating Sequence : simulink/Sources/Repeating Sequence  rep_seq_t=[0 0.00005 0.0001]  rep_seq_y=[-1 1 -1]
  PWM1 : Outport
  PWM2 : Outport  Port=2
  PWM3 : Outport  Port=3
  PWM4 : Outport  Port=4
  PWM5 : Outport  Port=5
  PWM6 : Outport  Port=6
  wires:
  Varef/1 -> Relational Operator/1
  Logical Operator2/1 -> PWM6/1
  Logical Operator1/1 -> PWM4/1
  Relational Operator2/1 -> PWM5/1, Logical Operator2/1
  Relational Operator1/1 -> PWM3/1, Logical Operator1/1
  Repeating Sequence/1 -> Relational Operator1/2, Relational Operator/2, Relational Operator2/2
  Relational Operator/1 -> PWM1/1, Logical Operator/1
  Vbref/1 -> Relational Operator1/1
  Logical Operator/1 -> PWM2/1
  Vcref/1 -> Relational Operator2/1
